simulink model "untitled1"  (R2020b)
settings: Solver=VariableStepAuto  StartTime=0.0  StopTime=10.0  RelTol=1e-3
settings Model: Creator=ANUJA  LastModifiedBy=ANUJA

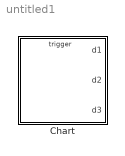
== system untitled1 ==
  Chart : Stateflow chart  TreatAsAtomicUnit=on

== stateflow chart untitled1/Chart ==
  state digit1 [parallel]
    settings: executionOrder=1
    state one
      en:d1=1;
    state two
      en:d1=2;
    state three
      en:d1=3;
    state four
      en:d1=4;
    state Zero
      en:d1=0;
    digit1.three -> digit1.four : inputclick
    Zero -> digit1.one : inputclick
    digit1.one -> digit1.two : inputclick
    digit1.two -> digit1.three : inputclick
    (default) -> Zero
    digit1.four -> Zero : inputclick/{digit2.inc2}
  state digit2 [parallel]
    settings: executionOrder=2
    state zero
      en:d2=0;
    state one
      en:d2=1;
    state two
      en:d2=2;
    state three
      en:d2=3;
    state four
      en:d2=4;
    digit2.one -> digit2.two : inc2
    digit2.two -> digit2.three : inc2
    digit2.three -> digit2.four : inc2
    (default) -> digit2.zero
    digit2.zero -> digit2.one : inc2
    digit2.four -> digit2.zero : inc2/{digit3.inc3}
  state digit3 [parallel]
    settings: executionOrder=3
    state zero
      en:d3=0;
    state one
      en:d3=1;
    state two
      en:d3=2;
    state three
      en:d3=3;
    state four
      en:d3=4;
    digit3.zero -> digit3.one : inc3
    digit3.one -> digit3.two : inc3
    digit3.two -> digit3.three : inc3
    digit3.three -> digit3.four : inc3
    (default) -> digit3.zero
    digit3.four -> digit3.zero : inc3
  data: d1 output; d2 output; d3 output
  events: inc2 local FUNCTION_CALL_EVENT; inc3 local FUNCTION_CALL_EVENT; inputclick input RISING_EDGE_EVENT
